simulink model "blockdemo"  (Simulink 6.3)
settings: Solver=FixedStepDiscrete  StartTime=0.0  StopTime=50  FixedStep=1  RelTol=1e-3
InitFcn:
  | %% DSPBuilder Start
  | alt_dspbuilder_update_model(bdroot)
  | %% DSPBuilder End
libraries: allblocks_alteradspbuilder2 x9, simulink x1
settings Model: Creator=mjervis  LastModifiedBy=delphick

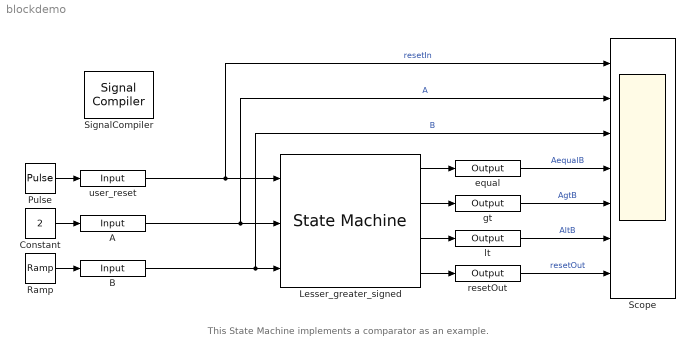
== system blockdemo ==
  note: This State Machine implements a comparator as an example.
  A : allblocks_alteradspbuilder2/Input  iofile=C:\workspace_clean\Documentation\DesignExamples\Tutorials\UnitBlocks\StateMachineFunctions\tb_blockdemo\blockdemo_A.salt  BusType=Signed Integer  bwl=3  bwr=0  SpecifyClock=off  PORTTYPE=Input
  B : allblocks_alteradspbuilder2/Input  iofile=C:\workspace_clean\Documentation\DesignExamples\Tutorials\UnitBlocks\StateMachineFunctions\tb_blockdemo\blockdemo_B.salt  BusType=Signed Integer  bwl=4  bwr=0  SpecifyClock=off  PORTTYPE=Input
  Constant : Constant  Value=2
  Lesser_greater_signed : allblocks_alteradspbuilder2/State Machine  Inputs=3  States=4  port_names=huh  parent_dir=C:\workspace_clean\Documentation\DesignExamples\Tutorials\UnitBlocks\StateMachineFunctions  db_dir=C:\workspace_clean\Documentation\DesignExamples\Tutorials\UnitBlocks\StateMachineFunctions\DSPBuilder_blockdemo  in_port1=reset  in_port2=A  in_port3=B  in_port4=reset  in_port5=reset  in_port6=reset  in_port7=reset  in_port8=reset  in_port9=reset  in_port10=reset  out_port1=equal  out_port2=A_gt_B  out_port3=A_lt_B  out_port4=rst  out_port5=equal  out_port6=equal  out_port7=equal  out_port8=equal  out_port9=equal  out_port10=equal  Outputs=4  db_entity=Lesser_greater_signed  table=1  inputs_edited=1110000000  outputs_edited=1111000000  VHDL_ARCHITECTURE=|
      | TYPE              
      | STATE_TYPE        
      | IS                
      | (equal_st,        
      | A_gt_B_st,        
      | A_lt_B_st,        
      | rst_st);          
      | SIGNAL            
      | current_state,    
      | next_state        
      | :                 
      | STATE_TYPE;       
      | SIGNAL            
      | reset_sig         
      | :                 
      | INTEGER;          
      | SIGNAL            
      | A_sig             
      | :                 
      | INTEGER;          
      | SIGNAL            
      | B_sig             
      | :                 
      | INTEGER;          
      | BEGIN             
      | reset_sig         
      | <=                
      | conv_integer      
      | (reset_input      
      | or                
      | aclr              
      | );                
      | A_sig             
      | <=                
      | conv_integer      
      | (                 
      | signed            
      | (input0)          
      | );                
      | B_sig             
      | <=                
      | conv_integer      
      | (                 
      | signed            
      | (input1)          
      | );                
      | PROCESS           
      | (clock,           
      | reset_sig)        
      | BEGIN             
      | IF                
      | (reset_sig=1)     
      | THEN              
      | current_state     
      | <=                
      | rst_st;           
      | ELSIF             
      | rising_edge(clock)
      | THEN              
      | current_state     
      | <=                
      | next_state;       
      | END               
      | IF;               
      | END               
      | PROCESS;          
      | PROCESS           
      | (current_state,   
      | A_sig,            
      | B_sig)            
      | BEGIN             
      | CASE              
      | current_state     
      | IS                
      | WHEN              
      | equal_st=>        
      | IF                
      | (A_sig>B_sig)     
      | THEN              
      | next_state        
      | <=                
      | A_gt_B_st;        
      | ELSIF             
      | (A_sig<B_sig)     
      | THEN              
      | next_state        
      | <=                
      | A_lt_B_st;        
      | ELSIF             
      | (A_sig=B_sig)     
      | THEN              
      | next_state        
      | <=                
      | equal_st;         
      | ELSE              
      | next_state        
      | <=                
      | equal_st;         
      | END               
      | IF;               
      | WHEN              
      | A_gt_B_st=>       
      | IF                
      | (A_sig=B_sig)     
      | THEN              
      | next_state        
      | <=                
      | equal_st;         
      | ELSIF             
      | (A_sig>B_sig)     
      | THEN              
      | next_state        
      | <=                
      | A_gt_B_st;        
      | ELSIF             
      | (A_sig<B_sig)     
      | THEN              
      | next_state        
      | <=                
      | A_lt_B_st;        
      | ELSE              
      | next_state        
      | <=                
      | A_gt_B_st;        
      | END               
      | IF;               
      | WHEN              
      | A_lt_B_st=>       
      | IF                
      | (A_sig=B_sig)     
      | THEN              
      | next_state        
      | <=                
      | equal_st;         
      | ELSIF             
      | (A_sig<B_sig)     
      | THEN              
      | next_state        
      | <=                
      | A_lt_B_st;        
      | ELSIF             
      | (A_sig>B_sig)     
      | THEN              
      | next_state        
      | <=                
      | A_gt_B_st;        
      | ELSE              
      | next_state        
      | <=                
      | A_lt_B_st;        
      | END               
      | IF;               
      | WHEN              
      | rst_st=>          
      | IF                
      | (A_sig=B_sig)     
      | THEN              
      | next_state        
      | <=                
      | equal_st;         
      | ELSIF             
      | (A_sig<B_sig)     
      | THEN              
      | next_state        
      | <=                
      | A_lt_B_st;        
      | ELSIF             
      | (A_sig>B_sig)     
      | THEN              
      | next_state        
      | <=                
      | A_gt_B_st;        
      | ELSE              
      | next_state        
      | <=                
      | rst_st;           
      | END               
      | IF;               
      | END               
      | CASE;             
      | END               
      | PROCESS;          
      | output1           
      | <=                
      | '1'               
      | WHEN              
      | current_state     
      | =                 
      | equal_st          
      | ELSE              
      | '0';              
      | output2           
      | <=                
      | '1'               
      | WHEN              
      | current_state     
      | =                 
      | A_gt_B_st         
      | ELSE              
      | '0';              
      | output3           
      | <=                
      | '1'               
      | WHEN              
      | current_state     
      | =                 
      | A_lt_B_st         
      | ELSE              
      | '0';              
      | output4           
      | <=                
      | '1'               
      | WHEN              
      | current_state     
      | =                 
      | rst_st            
      | ELSE              
      | '0';              
      | END               
      | a;
  Pulse : DiscretePulseGenerator  Period=100  PulseWidth=5
  Ramp : simulink/Sources/Ramp  slope=1  start=0  X0=0
  Scope : Scope  NumInputPorts=7
      settings: YMin=-0.5~-0.5~-10~-0.5~-0.5~-0.5~-0.5  YMax=1.5~2.5~10~1.5~1.5~1.5~1.5  SampleInput=on
  SignalCompiler : allblocks_alteradspbuilder2/Signal Compiler  DeviceFamily=Stratix IV  DeviceName=AUTO  EnableSignalTap=off  SignalTapDepth=128  UseBoardBlock=off  StpUseDefaultClock=on  StpClock=clock
  equal : allblocks_alteradspbuilder2/Output  iofile=C:\workspace_clean\Documentation\DesignExamples\Tutorials\UnitBlocks\StateMachineFunctions\tb_blockdemo\blockdemo_equal.capture  BusType=Single Bit  bwl=8  bwr=0  PORTTYPE=Output
  gt : allblocks_alteradspbuilder2/Output  iofile=C:\workspace_clean\Documentation\DesignExamples\Tutorials\UnitBlocks\StateMachineFunctions\tb_blockdemo\blockdemo_gt.capture  BusType=Single Bit  bwl=8  bwr=0  PORTTYPE=Output
  lt : allblocks_alteradspbuilder2/Output  iofile=C:\workspace_clean\Documentation\DesignExamples\Tutorials\UnitBlocks\StateMachineFunctions\tb_blockdemo\blockdemo_lt.capture  BusType=Single Bit  bwl=8  bwr=0  PORTTYPE=Output
  resetOut : allblocks_alteradspbuilder2/Output  iofile=C:\workspace_clean\Documentation\DesignExamples\Tutorials\UnitBlocks\StateMachineFunctions\tb_blockdemo\blockdemo_resetOut.capture  BusType=Single Bit  bwl=8  bwr=0  PORTTYPE=Output
  user_reset : allblocks_alteradspbuilder2/Input  iofile=C:\workspace_clean\Documentation\DesignExamples\Tutorials\UnitBlocks\StateMachineFunctions\tb_blockdemo\blockdemo_user_reset.salt  BusType=Single Bit  bwl=8  bwr=0  SpecifyClock=off  PORTTYPE=Input
  wires:
  user_reset/1 -> Lesser_greater_signed/1, Scope/1  "resetIn"
  A/1 -> Lesser_greater_signed/2, Scope/2  "A"
  B/1 -> Lesser_greater_signed/3, Scope/3  "B"
  Pulse/1 -> user_reset/1
  Lesser_greater_signed/1 -> equal/1
  Lesser_greater_signed/2 -> gt/1
  Lesser_greater_signed/3 -> lt/1
  Lesser_greater_signed/4 -> resetOut/1
  Ramp/1 -> B/1
  Constant/1 -> A/1
  equal/1 -> Scope/4  "AequalB"
  gt/1 -> Scope/5  "AgtB"
  lt/1 -> Scope/6  "AltB"
  resetOut/1 -> Scope/7  "resetOut"
